simulink model "simul2"  (R2021b)
settings: Solver=VariableStepAuto  StartTime=0.0  StopTime=10.0  RelTol=1e-3
settings Model: Creator=radek  LastModifiedBy=radek

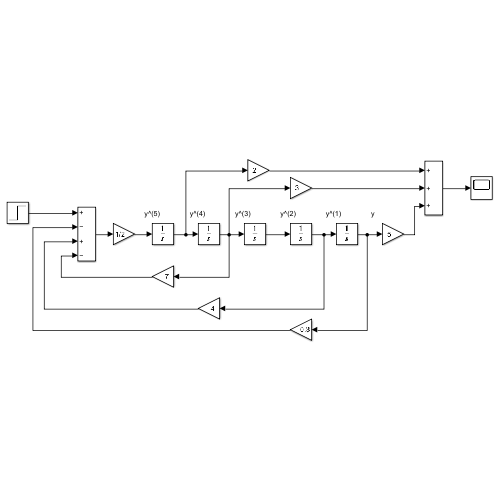
[thumbnail: Simulink's stored preview of the top-level diagram]
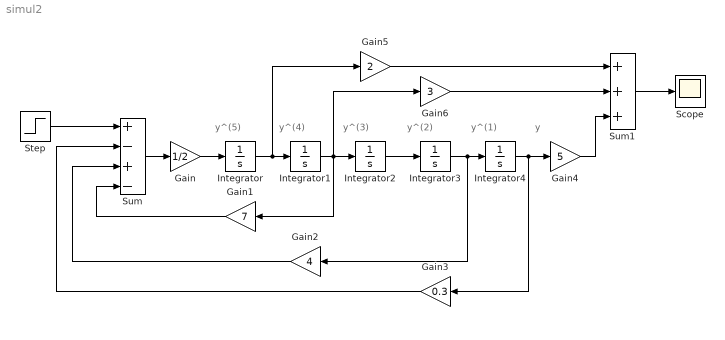
== system simul2 ==
  note: y
  note: y^(4)
  note: y^(5)
  note: y^(3)
  note: y^(2)
  note: y^(1)
  Gain : Gain  Gain=1/2
  Gain1 : Gain  Gain=7
  Gain2 : Gain  Gain=4
  Gain3 : Gain  Gain=0.3
  Gain4 : Gain  Gain=5
  Gain5 : Gain  Gain=2
  Gain6 : Gain  Gain=3
  Integrator{,1..4} (5 alike) : Integrator
  Scope : Scope
  Step : Step  SampleTime=0
  Sum : Sum  Inputs=+-+-
  Sum1 : Sum  Inputs=+++
  wires:
  Step/1 -> Sum/1
  Sum/1 -> Gain/1
  Integrator/1 -> Gain5/1, Integrator1/1
  Integrator3/1 -> Gain2/1, Integrator4/1
  Integrator4/1 -> Gain4/1, Gain3/1
  Gain1/1 -> Sum/4
  Gain2/1 -> Sum/3
  Gain3/1 -> Sum/2
  Gain4/1 -> Sum1/3
  Integrator2/1 -> Integrator3/1
  Sum1/1 -> Scope/1
  Gain5/1 -> Sum1/1
  Gain6/1 -> Sum1/2
  Integrator1/1 -> Gain1/1, Gain6/1, Integrator2/1
  Gain/1 -> Integrator/1
